simulink model "q20b"  (R2016a)
settings: Solver=VariableStepAuto  StartTime=0.0  StopTime=10.0  RelTol=1e-3
settings Model: Creator=Satya  LastModifiedBy=Satya

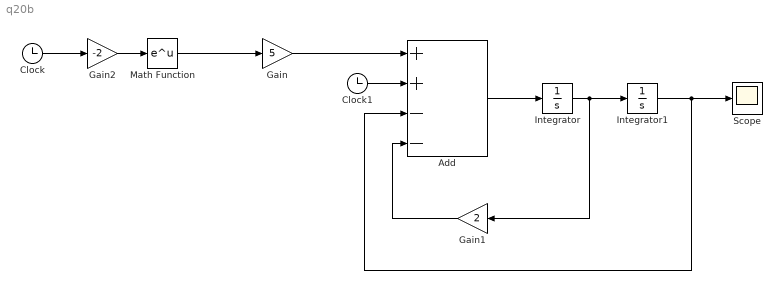
== system q20b ==
  Add : Sum  Inputs=++--
  Clock : Clock
  Clock1 : Clock
  Gain : Gain  Gain=5
  Gain1 : Gain  Gain=2
  Gain2 : Gain  Gain=-2
  Integrator : Integrator  InitialCondition=1
  Integrator1 : Integrator  InitialCondition=2
  Math Function : Math  SaturateOnIntegerOverflow=on
  Scope : Scope
  wires:
  Add/1 -> Integrator/1
  Integrator/1 -> Gain1/1, Integrator1/1
  Gain1/1 -> Add/4
  Integrator1/1 -> Add/3, Scope/1
  Clock1/1 -> Add/2
  Gain2/1 -> Math Function/1
  Clock/1 -> Gain2/1
  Math Function/1 -> Gain/1
  Gain/1 -> Add/1
